simulink model "robot_system_toolbox"  (R2021b)
settings: Solver=VariableStepAuto  StartTime=0.0  StopTime=0.5  RelTol=1e-3
undefined symbols (not defined in the file): eul2tform, initialConfig, targetPosition
libraries: robotmaniplib x15, robotcorelib x7
settings Model: Creator=tt006  LastModifiedBy=tt006

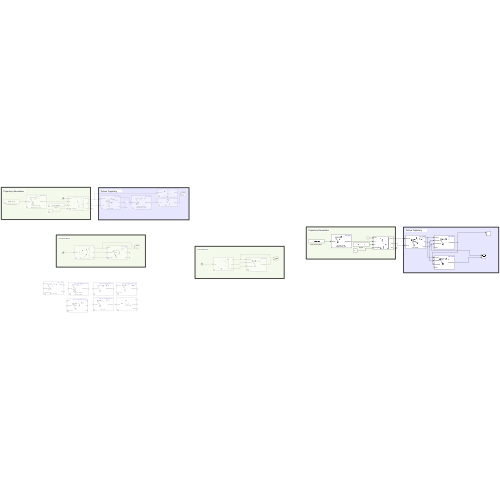
[thumbnail: Simulink's stored preview of the top-level diagram]
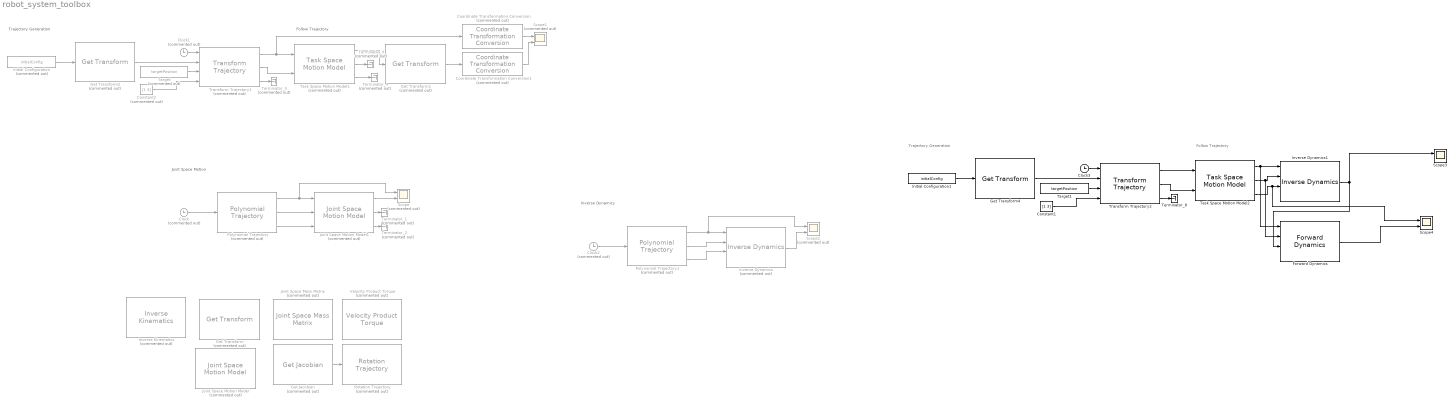
== system robot_system_toolbox ==
  note: Joint Space Motion
  note: Follow Trajectory
  note: Trajectory Generation
  note: Inverse Dynamics
  note: Follow Trajectory
  note: Trajectory Generation
  Clock : Clock  Commented=on
  Clock1 : Clock  Commented=on
  Clock2 : Clock  Commented=on
  Clock3 : Clock
  Constant1 : Constant  Value=[1 3]
  Constant2 : Constant  Commented=on  Value=[1 3]
  Coordinate Transformation Conversion : robotcorelib/Coordinate Transformation Conversion  Commented=on  InputRepresentation=Homogeneous Transformation  InputEulerSequence=ZYX  ShowTrVecInputPort=on  OutputRepresentation=Translation Vector  OutputEulerSequence=ZYX  ShowTrVecOutputPort=on  SimulateUsing=Interpreted execution
      settings: SourceProductBaseCode=NV,RO,RR,UV
  Coordinate Transformation Conversion1 : robotcorelib/Coordinate Transformation Conversion  Commented=on  InputRepresentation=Homogeneous Transformation  InputEulerSequence=ZYX  ShowTrVecInputPort=on  OutputRepresentation=Translation Vector  OutputEulerSequence=ZYX  ShowTrVecOutputPort=on  SimulateUsing=Interpreted execution
      settings: SourceProductBaseCode=NV,RO,RR,UV
  Forward Dynamics : robotmaniplib/Forward Dynamics  RigidBodyTree=ur5_robot  SimulateUsing=Interpreted execution
  Get Jacobian : robotmaniplib/Get Jacobian  Commented=on  RigidBodyTree=twoJointRigidBodyTree  EndEffector=tool  SimulateUsing=Interpreted execution
      settings: SourceProductBaseCode=RO
  Get Transform : robotmaniplib/Get Transform  Commented=on  RigidBodyTree=twoJointRigidBodyTree  SourceBody=base  TargetBody=base  SimulateUsing=Interpreted execution
  Get Transform1 : robotmaniplib/Get Transform  Commented=on  RigidBodyTree=ur5_robot  SourceBody=world  TargetBody=base_link  SimulateUsing=Interpreted execution
  Get Transform2 : robotmaniplib/Get Transform  Commented=on  RigidBodyTree=ur5_robot  SourceBody=world  TargetBody=base_link  SimulateUsing=Interpreted execution
  Get Transform4 : robotmaniplib/Get Transform  RigidBodyTree=ur5_robot  SourceBody=world  TargetBody=base_link  SimulateUsing=Interpreted execution
  Initial Configuration : Constant  Commented=on  Value=initialConfig  VectorParams1D=off  OutDataTypeStr=double
  Initial Configuration1 : Constant  Value=initialConfig  VectorParams1D=off  OutDataTypeStr=double
  Inverse Dynamics : robotmaniplib/Inverse Dynamics  Commented=on  RigidBodyTree=ur5_robot  SimulateUsing=Interpreted execution
      settings: SourceProductBaseCode=RO
  Inverse Dynamics1 : robotmaniplib/Inverse Dynamics  RigidBodyTree=ur5_robot  SimulateUsing=Interpreted execution
      settings: SourceProductBaseCode=RO
  Inverse Kinematics : robotmaniplib/Inverse Kinematics  Commented=on  RigidBodyTree=ur5_robot  EndEffector=ee_link  ShowInfo=on  SolverName=BFGS Gradient Projection  EnforceJointLimits=on  MaxIterations=1500  MaxTime=10  GradientTolerance=1e-7  SolutionTolerance=1e-6  StepTolerance=1e-14  ErrorChangeTolerance=1e-12  UseErrorDamping=on  DampingBias=0.0025  SimulateUsing=Interpreted execution
  Joint Space Mass Matrix : robotmaniplib/Joint Space Mass Matrix  Commented=on  RigidBodyTree=twoJointRigidBodyTree  SimulateUsing=Interpreted execution
  Joint Space Motion Model : robotmaniplib/Joint Space Motion Model  Commented=on  RigidBodyTree=twoJointRigidBodyTree  MotionType=Computed Torque Control  ProportionalGain=100  DerivativeGain=10  ErrorDynamicsSpecification=Damping Ratio / Natural Frequency  DampingRatio=1  NaturalFrequency=10  SettlingTime=0.59  Overshoot=0  ShowExternalForcePort=off  InitConfig=0  InitJointVel=0  SimulateUsing=Interpreted execution
      settings: SourceProductBaseCode=RO
  Joint Space Motion Model1 : robotmaniplib/Joint Space Motion Model  Commented=on  RigidBodyTree=ur5_robot  MotionType=Computed Torque Control  ProportionalGain=100  DerivativeGain=10  ErrorDynamicsSpecification=Damping Ratio / Natural Frequency  DampingRatio=1  NaturalFrequency=10  SettlingTime=0.59  Overshoot=0  ShowExternalForcePort=off  InitConfig=0  InitJointVel=0  SimulateUsing=Interpreted execution
      settings: SourceProductBaseCode=RO
  Polynomial Trajectory : robotcorelib/Polynomial Trajectory  Commented=on  WaypointSource=Internal  Waypoints=rand(6,5)  TimePoints=[ 0, 1, 2, 3, 4 ]  TimeInterval=[ 1, 4 ]  Method=Cubic Polynomial  ParameterSource=Internal  VelocityBoundaryCondition=zeros( 6, 5 )  AccelerationBoundaryCondition=zeros( 2, 5 )  SimulateUsing=Interpreted execution
  Polynomial Trajectory1 : robotcorelib/Polynomial Trajectory  Commented=on  WaypointSource=Internal  Waypoints=rand(6,5)  TimePoints=[ 0, 1, 2, 3, 4 ]  TimeInterval=[ 1, 4 ]  Method=Cubic Polynomial  ParameterSource=Internal  VelocityBoundaryCondition=zeros( 6, 5 )  AccelerationBoundaryCondition=zeros( 2, 5 )  SimulateUsing=Interpreted execution
  Rotation Trajectory : robotcorelib/Rotation Trajectory  Commented=on  WaypointFormat=Quaternion  WaypointSource=Internal  R0=[ 1, 0, 0, 0 ]'  RF=[ 0, 0, 1, 0 ]'  TimeInterval=[ 0, 1 ]  CustomTimeScaling=off  ParameterSource=Internal  TSTime=0:0.1:1  TimeScaling=[ 0:0.1:1; ones( 1, 11 ); zeros( 1, 11 ) ]  SimulateUsing=Interpreted execution
      settings: SourceProductBaseCode=NV,RO,RR,UV
  Scope : Scope  Commented=on  NumInputPorts=2
  Scope1 : Scope  Commented=on  NumInputPorts=2
  Scope2 : Scope  Commented=on  NumInputPorts=2
  Scope3 : Scope  NumInputPorts=2
  Scope4 : Scope  NumInputPorts=2
  Target : Constant  Commented=on  Value=targetPosition
  Target1 : Constant  Value=targetPosition
  Task Space Motion Model1 : robotmaniplib/Task Space Motion Model  Commented=on  RigidBodyTree=ur5_robot  EndEffector=tool0  ProportionalGain=700*eye(6)  DerivativeGain=350*eye(6)  JointDamping=1  ShowExternalForcePort=off  InitConfig=0  InitJointVel=0  SimulateUsing=Interpreted execution
      settings: SourceProductBaseCode=RO
  Task Space Motion Model2 : robotmaniplib/Task Space Motion Model  RigidBodyTree=ur5_robot  EndEffector=tool0  ProportionalGain=700*eye(6)  DerivativeGain=350*eye(6)  JointDamping=1  ShowExternalForcePort=off  InitConfig=0  InitJointVel=0  SimulateUsing=Interpreted execution
      settings: SourceProductBaseCode=RO
  Terminator_{1..5} (5 alike) : Terminator  Commented=on
  Terminator_8 : Terminator
  Transform Trajectory1 : robotcorelib/Transform Trajectory  Commented=on  WaypointSource=External  T0=getTra  TF=eul2tform( [ 0, pi, pi / 2 ] )  TimeInterval=[ 2, 3 ]  CustomTimeScaling=off  ParameterSource=Internal  TSTime=2:0.1:3  TimeScaling=[ 0:0.1:1; ones( 1, 11 ); zeros( 1, 11 ) ]  SimulateUsing=Interpreted execution
      settings: SourceProductBaseCode=NV,RO,RR,UV
  Transform Trajectory2 : robotcorelib/Transform Trajectory  WaypointSource=External  T0=getTra  TF=eul2tform( [ 0, pi, pi / 2 ] )  TimeInterval=[ 2, 3 ]  CustomTimeScaling=off  ParameterSource=Internal  TSTime=2:0.1:3  TimeScaling=[ 0:0.1:1; ones( 1, 11 ); zeros( 1, 11 ) ]  SimulateUsing=Interpreted execution
      settings: SourceProductBaseCode=NV,RO,RR,UV
  Velocity Product Torque : robotmaniplib/Velocity Product Torque  Commented=on  RigidBodyTree=twoJointRigidBodyTree  SimulateUsing=Interpreted execution
      settings: SourceProductBaseCode=RO
  wires:
  Polynomial Trajectory/2 -> Joint Space Motion Model1/2
  Joint Space Motion Model1/2 -> Terminator_1/1
  Polynomial Trajectory/1 -> Joint Space Motion Model1/1, Scope/1
  Clock/1 -> Polynomial Trajectory/1
  Joint Space Motion Model1/1 -> Scope/2
  Joint Space Motion Model1/3 -> Terminator_2/1
  Polynomial Trajectory/3 -> Joint Space Motion Model1/3
  Coordinate Transformation Conversion1/1 -> Scope1/2
  Transform Trajectory1/2 -> Task Space Motion Model1/2
  Task Space Motion Model1/1 -> Get Transform1/1
  Constant2/1 -> Transform Trajectory1/4
  Transform Trajectory1/3 -> Terminator_5/1
  Clock1/1 -> Transform Trajectory1/1
  Coordinate Transformation Conversion/1 -> Scope1/1
  Transform Trajectory1/1 -> Coordinate Transformation Conversion/1, Task Space Motion Model1/1
  Target/1 -> Transform Trajectory1/3
  Get Transform1/1 -> Coordinate Transformation Conversion1/1
  Task Space Motion Model1/2 -> Terminator_3/1
  Get Transform2/1 -> Transform Trajectory1/2
  Initial Configuration/1 -> Get Transform2/1
  Task Space Motion Model1/3 -> Terminator_4/1
  Inverse Dynamics/1 -> Scope2/2
  Polynomial Trajectory1/1 -> Inverse Dynamics/1, Scope2/1
  Polynomial Trajectory1/3 -> Inverse Dynamics/3
  Clock2/1 -> Polynomial Trajectory1/1
  Polynomial Trajectory1/2 -> Inverse Dynamics/2
  Transform Trajectory2/3 -> Terminator_8/1
  Initial Configuration1/1 -> Get Transform4/1
  Get Transform4/1 -> Transform Trajectory2/2
  Target1/1 -> Transform Trajectory2/3
  Transform Trajectory2/2 -> Task Space Motion Model2/2
  Constant1/1 -> Transform Trajectory2/4
  Clock3/1 -> Transform Trajectory2/1
  Transform Trajectory2/1 -> Task Space Motion Model2/1
  Get Jacobian/1 -> Rotation Trajectory/1
  Task Space Motion Model2/1 -> Forward Dynamics/1, Inverse Dynamics1/1
  Task Space Motion Model2/2 -> Forward Dynamics/2, Inverse Dynamics1/2
  Task Space Motion Model2/3 -> Scope4/1, Inverse Dynamics1/3
  Inverse Dynamics1/1 -> Forward Dynamics/3, Scope3/1
  Forward Dynamics/1 -> Scope4/2
